simulink model "dspwdnoisf"  (Simulink 5.0)
settings: Solver=FixedStepDiscrete  StartTime=0.0  StopTime=1024  RelTol=1e-3
PreLoadFcn:
  | load dspwlets;
values from neighbouring files (symbols this model uses):
  ts = [-1 0]    [lmsxy.m]    (also in sdspwwvdisp.m = get_param(blk,'CompiledSampleTime'))
undefined symbols (not defined in the file or in its folder): lod
libraries: dspsigattribs x8, dspsigops x3, dspsnks4 x3, dspmlti4 x2, dspsrcs4 x1
settings Model: Creator=don  LastModifiedBy=mkhan  ExtModeTrigMode=oneshot  ExtModeArmWhenConnect=off  SaveTime=off  SaveOutput=off  LimitDataPoints=off  SignalLoggingName=logsOut  IntegerOverflowMsg=none  RTWInlineParameters=on  BlockReductionOpt=off  BooleanDataType=off  ZeroCrossControl=UseLocalSettings  TargetHWChar=2  TargetHWWordLengths=8,16,32,32  RTWMathFcnLibMatFile=iso_c_tmw.mat  RTWOptions="-aEnforceIntegerDowncast=1 -aFoldNonRolledExpr=1 -aInlineInvariantSignals=1 -aInlineParameters=1 -aLocalBlockOutputs=1 -aRollThreshold=2 -aRTWVerbose=1 -aForceParamTrailComments=0 -aGenerateComments=1 -aIgnoreCustomStorageClasses=1 -aIncHierarchyInIds=0 -aMaxRTWIdLen=31 -aShowEliminatedStatements=0 -aReadOnly=0 -aTargetFcnLib=\"iso_c_tmw.mat\" -aIncDataTypeInIds=0 -aPrefixModelToSubsysFcnNames=1 -aInlinedPrmAccess=\"Literals\" -aGenerateFullHeader=1 -aIsPILTarget=0 -aGenerateReport=0 -aLogVarNameModifier=\"rt_\" -aExtMode=0 -aExtModeStaticAlloc=0 -aExtModeTesting=0 -aExtModeStaticAllocSize=1000000 -aExtModeTransport=0"

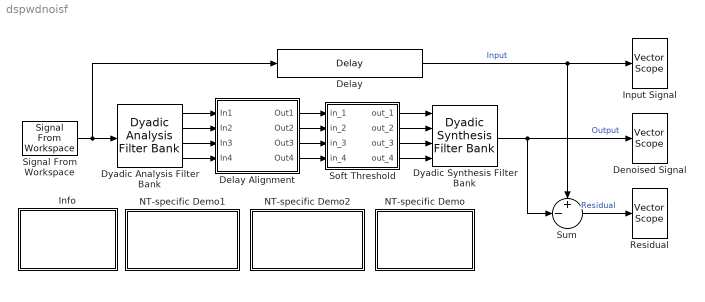
== system dspwdnoisf ==
  Delay : dspsigops/Delay  dly_unit=Samples  delay=7*(length(lod)-1)  ic_detail=on  dif_ic_for_ch=off  dif_ic_for_dly=off  ic=0  reset_popup=None
  Delay Alignment : Subsystem
  Denoised Signal : dspsnks4/Vector Scope  ScopeProperties=on  Domain=Time  HorizSpan=15  DisplayProperties=off  AxisGrid=on  Memory=off  FrameNumber=on  AxisLegend=off  AxisZoom=off  OpenScopeAtSimStart=on  OpenScopeImmediately=off  FigPos=[720 345 430 200]  AxisProperties=off  XUnits=Hertz  XRange=[0...Fs/2]  InheritXIncr=on  XIncr=1  XLabel=Samples  YUnits=dB  YLabel=Amplitude  LineProperties=off
      settings: YMin=-10  YMax=10
  Dyadic Analysis Filter Bank : dspmlti4/Dyadic Analysis Filter Bank  Wname=User-defined  OrdRec_ordDec=[1 / 1]  Order=2  LPF=lod  HPF=hid  NumLevels=3  tree=Asymmetric  Output=Multiple ports
  Dyadic Synthesis Filter Bank : dspmlti4/Dyadic Synthesis Filter Bank  Wname=User-defined  OrdRec_ordDec=[1 / 1]  Order=2  LPF=lor  HPF=hir  NumLevels=3  tree=Asymmetric  Input=Multiple ports
  Info : Subsystem
      mask Type: Frame-Based Simulation Info
      mask Display: disp('Info')
  Input Signal : dspsnks4/Vector Scope  ScopeProperties=on  Domain=Time  HorizSpan=15  DisplayProperties=off  AxisGrid=on  Memory=off  FrameNumber=on  AxisLegend=off  AxisZoom=off  OpenScopeAtSimStart=on  OpenScopeImmediately=off  FigPos=[720 590 430 200]  AxisProperties=off  XUnits=Hertz  XRange=[0...Fs/2]  InheritXIncr=on  XIncr=1  XLabel=Samples  YUnits=dB  YLabel=Amplitude  LineProperties=off
      settings: YMin=-10  YMax=10
  NT-specific Demo : Subsystem
      settings: OpenFcn=dspwdnoisf_win32
      mask Type: NT-only Demo
      mask Display: disp('PC/Windows\nDemo')
  NT-specific Demo1 : Subsystem
      settings: OpenFcn=dspwdnois
      mask Type: Sample-Based Demo
      mask Display: disp('Sample-Based\nDemo')
  NT-specific Demo2 : Subsystem
      settings: OpenFcn=dspwdnoisfp
      mask Type: Fixed-Point Demo
      mask Display: disp('Fixed-Point\nDemo')
  Residual : dspsnks4/Vector Scope  ScopeProperties=on  Domain=Time  HorizSpan=15  DisplayProperties=off  AxisGrid=on  Memory=off  FrameNumber=on  AxisLegend=off  AxisZoom=off  OpenScopeAtSimStart=on  OpenScopeImmediately=off  FigPos=[720 100 430 200]  AxisProperties=off  XUnits=Hertz  XRange=[0...Fs/2]  InheritXIncr=on  XIncr=1  XLabel=Samples  YUnits=dB  YLabel=Amplitude  LineProperties=off
      settings: YMin=-3.00160967239117  YMax=2.37514789840845
  Signal From Workspace : dspsrcs4/Signal From Workspace  X=noisdopp  Ts=ts  nsamps=64  OutputAfterFinalValue=Setting to zero
  Soft Threshold : Subsystem  mask(Soft Threshold){st=[3 2 1 0]}
      mask prompts: st "Vector of thresholds for each level:"
      mask help: Apply a soft threshold (deadzone transfer function) to each signal in the decomposition. First threshold applies to top-most filter bank output.
      mask init:
      | x=([-1 1 NaN 0 0 NaN -1 -.5 .5 1]+1)/2*.7+.15;
      | y=([0 0 NaN -1 1 NaN -1 0 0 1]+1)/2*.7+.05;
      mask Help: Vector of thresholds for each decomposition level.
      mask Display:
      | text(.1,.9,'Dead Zone')
      | plot(x,y)
  Sum : Sum  Inputs=+-|  SaturateOnIntegerOverflow=on  InputSameDT=on
  wires:
  Signal From Workspace/1 -> Dyadic Analysis Filter Bank/1, Delay/1
  Dyadic Analysis Filter Bank/4 -> Delay Alignment/4(In4)
  Dyadic Analysis Filter Bank/3 -> Delay Alignment/3(In3)
  Dyadic Analysis Filter Bank/2 -> Delay Alignment/2(In2)
  Dyadic Analysis Filter Bank/1 -> Delay Alignment/1(In1)
  Delay Alignment/4(Out4) -> Soft Threshold/4(in_4)
  Delay Alignment/3(Out3) -> Soft Threshold/3(in_3)
  Delay Alignment/2(Out2) -> Soft Threshold/2(in_2)
  Delay Alignment/1(Out1) -> Soft Threshold/1(in_1)
  Soft Threshold/1(out_1) -> Dyadic Synthesis Filter Bank/1
  Soft Threshold/2(out_2) -> Dyadic Synthesis Filter Bank/2
  Soft Threshold/3(out_3) -> Dyadic Synthesis Filter Bank/3
  Soft Threshold/4(out_4) -> Dyadic Synthesis Filter Bank/4
  Dyadic Synthesis Filter Bank/1 -> Sum/2, Denoised Signal/1  "Output"
  Sum/1 -> Residual/1  "Residual"
  Delay/1 -> Sum/1, Input Signal/1  "Input"

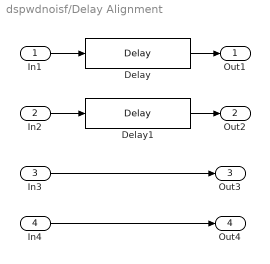
== system dspwdnoisf/Delay Alignment ==
  In1 : Inport
  In2 : Inport  Port=2
  In3 : Inport  Port=3
  In4 : Inport  Port=4
  Delay : dspsigops/Delay  dly_unit=Samples  delay=3*(length(lod)-1)  ic_detail=on  dif_ic_for_ch=off  dif_ic_for_dly=off  ic=0  reset_popup=None
  Delay1 : dspsigops/Delay  dly_unit=Samples  delay=length(lod) - 1  ic_detail=on  dif_ic_for_ch=off  dif_ic_for_dly=off  ic=0  reset_popup=None
  Out1 : Outport
  Out2 : Outport  Port=2
  Out3 : Outport  Port=3
  Out4 : Outport  Port=4
  wires:
  In3/1 -> Out3/1
  In4/1 -> Out4/1
  In2/1 -> Delay1/1
  Delay1/1 -> Out2/1
  In1/1 -> Delay/1
  Delay/1 -> Out1/1

== system dspwdnoisf/Info ==
  note: Demonstration of wavelet de-noising
      |
      |
      | Set the threshold levels in the "Soft Threshold" block
      | to alter the de-noising characteristics of the system:
      |
      | Threshold=[0 0 0 0]  -> No de-noising
      | (perfect reconstruction)
      |
      | Threshold=[3 2 1 0] -> Moderate de-noising
      | (removes small-scale content from signal)

== system dspwdnoisf/NT-specific Demo ==

== system dspwdnoisf/NT-specific Demo1 ==

== system dspwdnoisf/NT-specific Demo2 ==

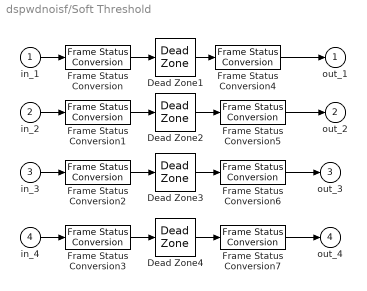
== system dspwdnoisf/Soft Threshold ==
  in_1 : Inport
  in_2 : Inport  Port=2
  in_3 : Inport  Port=3
  in_4 : Inport  Port=4
  Dead Zone1 : DeadZone  LowerValue=-st(1)  UpperValue=st(1)  ZeroCross=off  SaturateOnIntegerOverflow=on
  Dead Zone2 : DeadZone  LowerValue=-st(2)  UpperValue=st(2)  ZeroCross=off  SaturateOnIntegerOverflow=on
  Dead Zone3 : DeadZone  LowerValue=-st(3)  UpperValue=st(3)  ZeroCross=off  SaturateOnIntegerOverflow=on
  Dead Zone4 : DeadZone  LowerValue=-st(4)  UpperValue=st(4)  ZeroCross=off  SaturateOnIntegerOverflow=on
  Frame Status Conversion{,1..3} (4 alike) : dspsigattribs/Frame Status Conversion  growRefPort=off  outframe=Sample-based
  Frame Status Conversion{4..7} (4 alike) : dspsigattribs/Frame Status Conversion  growRefPort=off  outframe=Frame-based
  out_1 : Outport  InitialOutput=0
  out_2 : Outport  Port=2  InitialOutput=0
  out_3 : Outport  Port=3  InitialOutput=0
  out_4 : Outport  Port=4  InitialOutput=0
  wires:
  in_1/1 -> Frame Status Conversion/1
  Frame Status Conversion/1 -> Dead Zone1/1
  in_2/1 -> Frame Status Conversion1/1
  Frame Status Conversion1/1 -> Dead Zone2/1
  in_3/1 -> Frame Status Conversion2/1
  Frame Status Conversion2/1 -> Dead Zone3/1
  in_4/1 -> Frame Status Conversion3/1
  Frame Status Conversion3/1 -> Dead Zone4/1
  Dead Zone1/1 -> Frame Status Conversion4/1
  Frame Status Conversion4/1 -> out_1/1
  Dead Zone2/1 -> Frame Status Conversion5/1
  Frame Status Conversion5/1 -> out_2/1
  Dead Zone3/1 -> Frame Status Conversion6/1
  Frame Status Conversion6/1 -> out_3/1
  Dead Zone4/1 -> Frame Status Conversion7/1
  Frame Status Conversion7/1 -> out_4/1
